simulink model "v00_0A_0E"  (R2022b)
settings: Solver=FixedStepDiscrete  StartTime=0.0  StopTime=8000  FixedStep=SampleTime  MaxStep=Contactors_StepTime_msec  RelTol=1e-3  EnableMultiTasking=on
undefined symbols (not defined in the file): A_to_mA, BalancingTempGroup, canChannel, CapacityFactor, CC_Inputs, CellSOC, ChargeState, ContactorsFlags, DiscIntNeverNeededParam, gEN_Contactors_StepTime_msec, Ion, isDynamicCurrentEn, Lithium, maxAllowedImbalance, nCells_parallel, nCells_series, nCellTempGrps, PermanentFailRecoveryTrigger, ProtectionFlags, RBal_ohm, SampleTime, sigbuilder_block, StLineEq_varA, StLineEq_varB, TempSelectForDCL, Thresholds, V_to_mV
libraries: simulink x32, spsIdealSwitchLib x21, spsBatteryLib x20, spsSeriesRLCBranchLib x20, spsVoltageMeasurementLib x20, canmsglib x4, canlib x3, dspstat3 x2, spspowerguiLib x2, spsControlledCurrentSourceLib x1, spsCurrentMeasurementLib x1
(part 5 of 7)

== stateflow chart v00_0A_0E/Contactors/Contactor_StateMachine ==
  settings: sampleTime=Contactors_StepTime_msec
  state ContactorOperations
    state Open_Substate
      en:
      NegContactors = ContactorsFlags.Open;
      PosContactors = ContactorsFlags.Open;
      PreChargeContactors = ContactorsFlags.Open;
      ContactorsWeldWarning = ContactorsFlags.None;
      ContactorsState = ContState.OpenSubstate;
    note: Set contactor fault flag to weld
    note: Configurable limit to ContWeldCheckLimit
        | previously set to '5'
    state IntState9
      en:
    note: Added External Short Circuit Detection and Counter Logic
    note: Reattempt precharge. Return to start to stabilize, verify if it should close, etc
    state PreCharging_Substate_Old
      state NegContact_Check
        entry:
        NegContactors = ContactorsFlags.Closed;
        ContactorsState = ContState.PreCharging_NegContactorClosed;
      state IntState10
        en:
      state IntState9
        en:
      state ChangeState01_to_Opening
      state PreCharge_Check01
        entry:PreTimeReset=1;
        PreChargeContactors = ContactorsFlags.Closed;
        ContactorsState = ContState.PreCharging_PreChargeClosed;
      state IntState11
        en:
      state IntState13
        en:
      state IntState12
        en:
      state IntState16
        en:
      state IntState15
        en:
      state PreCharge_Check03
        en:
        PreChargeContactors = ContactorsFlags.Open;
        ContactorsState = ContState.PreCharging_PreChargeRetry;
      state PosContact_Check
        entry:
        PosContactors = ContactorsFlags.Closed;
        ContactorsState = ContState.PreCharging_PosContactorClosed;
      state IntState14
        en:
      state PreCharge_Check02
        entry:
        PreChargeContactors = ContactorsFlags.Open;
        ContactorsState = ContState.PreCharging_PreChargeOpen;
      ContactorOperations.PreCharging_Substate_Old.NegContact_Check -> IntState10 [order 2] : [NegContactors_FB == 0]{PreTimeReset=1;}
      IntState10 -> ContactorOperations.PreCharging_Substate_Old.NegContact_Check [order 2] : [NegContactors_FB == 1]{PreTimeReset=0;}
      ContactorOperations.PreCharging_Substate_Old.IntState9 -> ContactorOperations.PreCharging_Substate_Old.NegContact_Check [order 2] : [NegContactors_FB == 0 || BMS_State==4]{PreTimeReset=0;}
      ContactorOperations.PreCharging_Substate_Old.NegContact_Check -> ContactorOperations.PreCharging_Substate_Old.IntState9 [order 1] : [NegContactors_FB == 1 && BMS_State~=4]{PreTimeReset = 1;}
      IntState10 -> ContactorOperations.PreCharging_Substate_Old.ChangeState01_to_Opening [order 1] : [PreIntegratedTime>Thresholds.ContCutoffTime_msec]{PreTimeReset=0;}
      ContactorOperations.PreCharging_Substate_Old.IntState9 -> ContactorOperations.PreCharging_Substate_Old.PreCharge_Check01 [order 1] : [PreIntegratedTime>Thresholds.ContCutoffTime_msec]{PreTimeReset=0;}
      ContactorOperations.PreCharging_Substate_Old.PreCharge_Check01 -> IntState11 [order 3] : [PreChargeContactors_FB ==0]{PreTimeReset=1;}
      IntState11 -> ContactorOperations.PreCharging_Substate_Old.ChangeState01_to_Opening [order 1] : [PreIntegratedTime>Thresholds.ContCutoffTime_msec]{PreTimeReset=0;}
      IntState11 -> ContactorOperations.PreCharging_Substate_Old.PreCharge_Check01 [order 2] : [PreChargeContactors_FB ==1]{PreTimeReset=0;}
      ContactorOperations.PreCharging_Substate_Old.IntState16 -> ContactorOperations.PreCharging_Substate_Old.ChangeState01_to_Opening [order 1] : [PreIntegratedTime>Thresholds.ContCutoffTime_msec]{PreTimeReset=0;}
      ContactorOperations.PreCharging_Substate_Old.IntState15 -> ContactorOperations.PreCharging_Substate_Old.ChangeState01_to_Opening [order 1] : [PreIntegratedTime>Thresholds.ContCutoffTime_msec]
      ContactorOperations.PreCharging_Substate_Old.PreCharge_Check01 -> IntState13 [order 1] : [abs(DataPipeline.Current_mA) <= Thresholds.ContCurrent_mA]{PreTimeReset=1;}
      IntState13 -> ContactorOperations.PreCharging_Substate_Old.PreCharge_Check01 [order 2] : [abs(DataPipeline.Current_mA) > Thresholds.ContCurrent_mA]{PreTimeReset=0;}
      ContactorOperations.PreCharging_Substate_Old.PreCharge_Check01 -> ContactorOperations.PreCharging_Substate_Old.PreCharge_Check03 [order 2] : [PreIntegratedTime>Thresholds.PreChargeRetryTimeout_msec]{PreChargeRetryCheck = PreChargeRetryCheck + 1;PreTimeReset=0;}
      IntState12 -> ContactorOperations.PreCharging_Substate_Old.PreCharge_Check01 [order 1] : [PreIntegratedTime>Thresholds.PreChargeRecoveryTimeout_msec]{PreTimeReset=0;}
      IntState13 -> ContactorOperations.PreCharging_Substate_Old.PosContact_Check [order 1] : [PreIntegratedTime>Thresholds.PreChargeTimeout_msec]{PreTimeReset=0;}
      ContactorOperations.PreCharging_Substate_Old.PreCharge_Check03 -> IntState12 [order 2] : [PreChargeRetryCheck <= Thresholds.PreChargeRetryLimit]{PreTimeReset=1;}
      IntState12 -> ContactorOperations.PreCharging_Substate_Old.PreCharge_Check03 [order 2] : [PreChargeRetryCheck > Thresholds.PreChargeRetryLimit]{PreTimeReset=0;}
      ContactorOperations.PreCharging_Substate_Old.PreCharge_Check02 -> ContactorOperations.PreCharging_Substate_Old.IntState16 [order 2] : [PreChargeContactors_FB ==1]{PreTimeReset=1;}
      ContactorOperations.PreCharging_Substate_Old.IntState16 -> ContactorOperations.PreCharging_Substate_Old.PreCharge_Check02 [order 2] : [PreChargeContactors_FB ==0]{PreTimeReset=0;}
      ContactorOperations.PreCharging_Substate_Old.PosContact_Check -> ContactorOperations.PreCharging_Substate_Old.IntState15 [order 1] : [PosContactors_FB == 0]{PreTimeReset=1;}
      ContactorOperations.PreCharging_Substate_Old.IntState15 -> ContactorOperations.PreCharging_Substate_Old.PosContact_Check [order 2] : [PosContactors_FB == 0]{PreTimeReset=0;}
      ContactorOperations.PreCharging_Substate_Old.PosContact_Check -> ContactorOperations.PreCharging_Substate_Old.IntState14 [order 2] : [PosContactors_FB == 1]{PreTimeReset=1;}
      ContactorOperations.PreCharging_Substate_Old.IntState14 -> ContactorOperations.PreCharging_Substate_Old.PosContact_Check [order 2] : [PosContactors_FB == 0]{PreTimeReset=0;}
      ContactorOperations.PreCharging_Substate_Old.IntState14 -> ContactorOperations.PreCharging_Substate_Old.PreCharge_Check02 [order 1] : [PreIntegratedTime>Thresholds.ContCutoffTime_msec]{PreTimeReset=0;}
    state IntState
      en:
    state Permanent_Fail [group]
      state PermanentFail
        entry:
        NegContactors = ContactorsFlags.Open;
        PosContactors = ContactorsFlags.Open;
        PreChargeContactors = ContactorsFlags.Open;
        PermanentFail = ProtectionFlags.Error;
        ContactorsState = ContState.PermanentFailure;
    state PreCharging_Substate_New
      state NegContact_Check
        en:
        NegContactors = ContactorsFlags.Closed;
        ContactorsState = ContState.PreCharging_NegContactorClosed;
      state IntState1
        en:
      state IntState4
        en:
      state PreCharge_Check01
        en: PreTimeReset = 1;
        PreChargeContactors = ContactorsFlags.Closed;
        ContactorsState = ContState.PreCharging_PreChargeClosed;
      state ChangeState01_to_Opening
      state IntState5
        en:
      state IntState3
        en:
      state IntState2
        en:
      state PreCharge_Check03
        en: PreTimeReset=1;
        PreChargeContactors = ContactorsFlags.Open;
        ContactorsState = ContState.PreCharging_PreChargeRetry;
      state IntState7
        en:
      state IntState6
        en:
      state PosContact_Check
        en:
        PosContactors = ContactorsFlags.Closed;
        ContactorsState = ContState.PreCharging_PosContactorClosed;
      state IntState8
        en:
      state PreCharge_Check02
        en:
        PreChargeContactors = ContactorsFlags.Open;
        ContactorsState = ContState.PreCharging_PreChargeOpen;
      ContactorOperations.PreCharging_Substate_New.NegContact_Check -> IntState4 [order 1] : [NegContactors_FB == 0]{PreTimeReset=1;}
      IntState4 -> ContactorOperations.PreCharging_Substate_New.NegContact_Check [order 2] : [NegContactors_FB==1]{PreTimeReset=0;}
      IntState1 -> ContactorOperations.PreCharging_Substate_New.NegContact_Check [order 1] : [NegContactors_FB == 0]{PreTimeReset=0;}
      ContactorOperations.PreCharging_Substate_New.NegContact_Check -> IntState1 [order 2] : [NegContactors_FB == 1]{PreTimeReset = 1;}
      IntState1 -> ContactorOperations.PreCharging_Substate_New.PreCharge_Check01 [order 2] : [PreIntegratedTime>Thresholds.ContCutoffTime_msec]{PreTimeReset=0;}
      IntState4 -> ContactorOperations.PreCharging_Substate_New.ChangeState01_to_Opening [order 1] : [PreIntegratedTime>Thresholds.ContCutoffTime_msec]{PreTimeReset=0;}
      ContactorOperations.PreCharging_Substate_New.PreCharge_Check01 -> IntState5 [order 1] : [PreChargeContactors_FB ==0]{PreTimeReset=1;}
      IntState5 -> ContactorOperations.PreCharging_Substate_New.PreCharge_Check01 [order 2] : [PreChargeContactors_FB==1]{PreTimeReset=0;}
      ContactorOperations.PreCharging_Substate_New.PreCharge_Check01 -> IntState3 [order 2] : [abs(DataPipeline.Current_mA) < Thresholds.PreChargeEndMaxCurrent_mA && VoltageDelta_mV < Thresholds.PreChargeVoltageDelta_mV]{PreTimeReset=1;}
      IntState3 -> ContactorOperations.PreCharging_Substate_New.PreCharge_Check01 [order 2] : [abs(DataPipeline.Current_mA) > Thresholds.PreChargeEndMaxCurrent_mA || VoltageDelta_mV > Thresholds.PreChargeVoltageDelta_mV]{PreTimeReset=0;}
      ContactorOperations.PreCharging_Substate_New.PreCharge_Check01 -> ContactorOperations.PreCharging_Substate_New.PreCharge_Check03 [order 3] : [PreIntegratedTime>Thresholds.PreChargeRetryTimeout_msec]{PreChargeRetryCheck = PreChargeRetryCheck + 1; PreTimeReset=0;}
      IntState2 -> ContactorOperations.PreCharging_Substate_New.PreCharge_Check01 [order 1] : [PreIntegratedTime>Thresholds.PreChargeRecoveryTimeout_msec]{PreTimeReset=0}
      IntState5 -> ContactorOperations.PreCharging_Substate_New.ChangeState01_to_Opening [order 1] : [PreIntegratedTime>Thresholds.ContCutoffTime_msec]{PreTimeReset=0;}
      IntState7 -> ContactorOperations.PreCharging_Substate_New.ChangeState01_to_Opening [order 1] : [PreIntegratedTime>Thresholds.ContCutoffTime_msec]{PreTimeReset=0;}
      IntState6 -> ContactorOperations.PreCharging_Substate_New.ChangeState01_to_Opening [order 1] : [PreIntegratedTime>Thresholds.ContCutoffTime_msec]{PreTimeReset=0;}
      IntState3 -> ContactorOperations.PreCharging_Substate_New.PosContact_Check [order 1] : [PreIntegratedTime>Thresholds.PreChargeTimeout_msec]{PreTimeReset=0;}
      ContactorOperations.PreCharging_Substate_New.PreCharge_Check03 -> IntState2 [order 2] : [PreChargeRetryCheck <= Thresholds.PreChargeRetryLimit]{PreTimeReset=1;}
      IntState2 -> ContactorOperations.PreCharging_Substate_New.PreCharge_Check03 [order 2] : [PreChargeRetryCheck > Thresholds.PreChargeRetryLimit]
      ContactorOperations.PreCharging_Substate_New.PreCharge_Check02 -> IntState7 [order 2] : [PreChargeContactors_FB ==1]{PreTimeReset=1;}
      IntState7 -> ContactorOperations.PreCharging_Substate_New.PreCharge_Check02 [order 2] : [PreChargeContactors_FB==0]{PreTimeReset=0;}
      IntState6 -> ContactorOperations.PreCharging_Substate_New.PosContact_Check [order 2] : [PosContactors_FB == 1]{PreTimeReset=0;}
      ContactorOperations.PreCharging_Substate_New.PosContact_Check -> IntState6 [order 2] : [PosContactors_FB == 0]{PreTimeReset=1;}
      ContactorOperations.PreCharging_Substate_New.PosContact_Check -> ContactorOperations.PreCharging_Substate_New.IntState8 [order 1] : [PosContactors_FB == 1]{PreTimeReset=1;}
      ContactorOperations.PreCharging_Substate_New.IntState8 -> ContactorOperations.PreCharging_Substate_New.PosContact_Check [order 2] : [PosContactors_FB==0]{PreTimeReset=0;}
      ContactorOperations.PreCharging_Substate_New.IntState8 -> ContactorOperations.PreCharging_Substate_New.PreCharge_Check02 [order 1] : [PreIntegratedTime>Thresholds.ContCutoffTime_msec]{PreTimeReset=0;}
    state IntState15
      en:
    state IntState16
      en:
    state Opening_Substate [group]
      state NegContact_Check_02
        en:
        NegContactors = ContactorsFlags.Open;
        PosContactors = ContactorsFlags.Open;
        ContactorsState = ContState.OpeningSubstate;
    state IntState14
      en:
    state IntState8
      en:
    state Closed_Substate
      en:
      NegContactors = ContactorsFlags.Closed;
      PosContactors = ContactorsFlags.Closed;
      PreChargeContactors = ContactorsFlags.Open;
      ContactorsWeldWarning = ContactorsFlags.None
      ContactorsState = ContState.ClosedSubstate;
    PermanentFail -> Open_Substate : [PermanentFailRecoveryTrigger == 1]{PreChargeRetryCheck=0}
    (default) -> Open_Substate
    Open_Substate -> PermanentFail [order 2] : [ProtectionOutput.ThermalRunaway== ProtectionFlags.Error|| ProtectionOutput.ShortCircuitDetect== ProtectionFlags.Error || DataPipeline.VCU.EmergencyDisconnectEn==1]
    ContactorOperations.IntState9 -> Open_Substate [order 2] : [Flags_detection==0 || DataPipeline.PreChargeLogic==1]{PreTimeReset=0;}
    Open_Substate -> ContactorOperations.IntState9 [order 3] : [Flags_detection == 1 && DataPipeline.PreChargeLogic == 0]{PreTimeReset=1;}
    ContactorOperations.IntState9 -> ContactorOperations.PreCharging_Substate_Old.NegContact_Check [order 1] : [PreIntegratedTime>Thresholds.OpenToPreChargeStateTime_msec]{PreTimeReset=0;}
    NegContact_Check_02 -> Open_Substate
    IntState -> Open_Substate [order 2] : [Flags_detection == 0 || DataPipeline.PreChargeLogic == 0]{PreTimeReset=0;}
    Open_Substate -> IntState [order 1] : [Flags_detection == 1 && DataPipeline.PreChargeLogic == 1]{PreTimeReset = 1;}
    IntState -> ContactorOperations.PreCharging_Substate_New.NegContact_Check [order 1] : [PreIntegratedTime>Thresholds.OpenToPreChargeStateTime_msec]{PreTimeReset=0;}
    ContactorOperations.PreCharging_Substate_Old.ChangeState01_to_Opening -> NegContact_Check_02
    ContactorOperations.PreCharging_Substate_Old.PreCharge_Check03 -> ContactorOperations.IntState15 [order 1] : [PreChargeRetryCheck > Thresholds.PreChargeRetryLimit]{PreTimeReset=1;}
    ContactorOperations.IntState15 -> PermanentFail [order 1] : [PreIntegratedTime>Thresholds.PreChargeTimeout_msec]{PreTimeReset=0;}
    ContactorOperations.IntState15 -> ContactorOperations.PreCharging_Substate_Old.PreCharge_Check03 [order 2] : [PreChargeRetryCheck < Thresholds.PreChargeRetryLimit]{PreTimeReset=0;}
    PreCharging_Substate_Old -> PermanentFail [order 1] : [ProtectionOutput.ThermalRunaway== ProtectionFlags.Error|| ProtectionOutput.ShortCircuitDetect== ProtectionFlags.Error || DataPipeline.VCU.EmergencyDisconnectEn==1]
    ContactorOperations.PreCharging_Substate_New.ChangeState01_to_Opening -> NegContact_Check_02
    ContactorOperations.PreCharging_Substate_Old.PreCharge_Check02 -> ContactorOperations.IntState14 [order 1] : [PreChargeContactors_FB == 0]{PreTimeReset=1;}
    ContactorOperations.IntState14 -> ContactorOperations.PreCharging_Substate_Old.PreCharge_Check02 [order 2] : [PreChargeContactors_FB == 1]{PreTimeReset=0;}
    PreCharging_Substate_Old -> NegContact_Check_02 [order 2] : [duration(Flags_detection == 0,msec) > Thresholds.PreToOpeningSubstate_msec]
    ContactorOperations.IntState16 -> ContactorOperations.PreCharging_Substate_New.PreCharge_Check03 [order 2] : [PreChargeRetryCheck < Thresholds.PreChargeRetryLimit]{PreTimeReset=0;}
    ContactorOperations.IntState16 -> PermanentFail [order 1] : [PreIntegratedTime>Thresholds.PreChargeTimeout_msec]{PreTimeReset=0;}
    ContactorOperations.PreCharging_Substate_New.PreCharge_Check03 -> ContactorOperations.IntState16 [order 1] : [PreChargeRetryCheck > Thresholds.PreChargeRetryLimit]{PreTimeReset=1;}
    PreCharging_Substate_New -> PermanentFail [order 2] : [ProtectionOutput.ThermalRunaway== ProtectionFlags.Error|| ProtectionOutput.ShortCircuitDetect== ProtectionFlags.Error || DataPipeline.VCU.EmergencyDisconnectEn==1]
    PreCharging_Substate_New -> NegContact_Check_02 [order 1] : [duration(Flags_detection == 0,msec) > Thresholds.PreToOpeningSubstate_msec]
    Closed_Substate -> NegContact_Check_02 [order 2] : [duration(Flags_detection == 0, msec) > Thresholds.FlagDebounceTime_msec]
    Closed_Substate -> PermanentFail [order 1] : [ProtectionOutput.ThermalRunaway== ProtectionFlags.Error|| ProtectionOutput.ShortCircuitDetect== ProtectionFlags.Error || DataPipeline.VCU.EmergencyDisconnectEn==1]
    ContactorOperations.IntState14 -> Closed_Substate [order 1] : [PreIntegratedTime>Thresholds.PreToClosed_Time_msec]{PreTimeReset=0;}
    ContactorOperations.PreCharging_Substate_New.PreCharge_Check02 -> ContactorOperations.IntState8 [order 1] : [PreChargeContactors_FB == 0]{PreTimeReset=1;}
    ContactorOperations.IntState8 -> ContactorOperations.PreCharging_Substate_New.PreCharge_Check02 [order 2] : [PreChargeContactors_FB==1]{PreTimeReset=0;}
    ContactorOperations.IntState8 -> Closed_Substate [order 1] : [PreIntegratedTime>Thresholds.PreToClosed_Time_msec]{PreTimeReset=0;}
  data: PreTimeReset output; PreIntegratedTime input; VoltageDelta_mV input; Flags_detection input; Thresholds input; DataPipeline input; NegContactors output Enum: ContactorsFlags =ContactorsFlags.Open; PosContactors output Enum: ContactorsFlags =ContactorsFlags.Open; PreChargeContactors output Enum: ContactorsFlags =ContactorsFlags.Open; NegContactors_FB input Enum: ContactorsFlags; PreChargeContactors_FB input Enum: ContactorsFlags; PosContactors_FB input Enum: ContactorsFlags; ContactorsWeldWarning output; PermanentFail output; PermanentFailRecoveryTrigger input; ContactorsState output Enum: ContState =ContState.OpenSubstate; ProtectionOutput input; PreChargeRetryCheck local =uint8(0); BMS_State input
